simulink model "schemaSimulink"  (R2022b)
settings: Solver=FixedStepAuto  StartTime=0.0  StopTime=10.0  FixedStep=1/60  RelTol=1e-3
undefined symbols (not defined in the file): beta, g, I, l, m
settings Model: Creator=giova  LastModifiedBy=giova

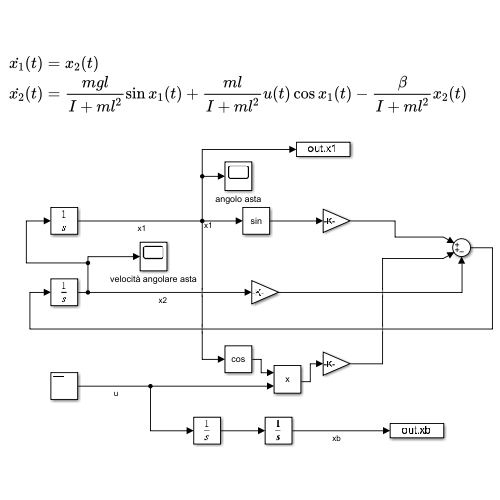
[thumbnail: Simulink's stored preview of the top-level diagram]
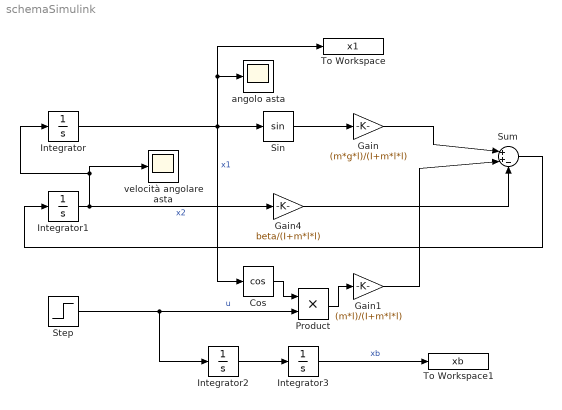
== system schemaSimulink ==
  Cos : Trigonometry  Operator=cos
  Gain : Gain  Gain=(m*g*l)/(I+m*l*l)
  Gain1 : Gain  Gain=(m*l)/(I+m*l*l)
  Gain4 : Gain  Gain=beta/(I+m*l*l)
  Integrator{,1..3} (4 alike) : Integrator
  Product : Product
  Sin : Trigonometry
  Step : Step  Time=0.1  Before=1  After=0  SampleTime=0
  Sum : Sum  Inputs=|++-
  To Workspace : ToWorkspace  VariableName=x1  SaveFormat=Timeseries  SampleTime=-1
  To Workspace1 : ToWorkspace  VariableName=xb  SaveFormat=Timeseries  SampleTime=-1
  angolo asta : Scope
  velocità angolare asta : Scope
  wires:
  Integrator1/1 -> Gain4/1, velocità angolare asta/1, Integrator/1  "x2"
  Integrator/1 -> Cos/1, angolo asta/1, To Workspace/1, Sin/1  "x1"
  Sin/1 -> Gain/1
  Cos/1 -> Product/1
  Step/1 -> Product/2, Integrator2/1  "u"
  Product/1 -> Gain1/1
  Gain/1 -> Sum/1
  Gain1/1 -> Sum/2
  Sum/1 -> Integrator1/1
  Integrator2/1 -> Integrator3/1
  Gain4/1 -> Sum/3
  Integrator3/1 -> To Workspace1/1  "xb"
